simulink model "ControladorEmbebido"  (R2022b)
settings: Solver=FixedStepDiscrete  StartTime=0.0  StopTime=SIMULPARAM.T_end  FixedStep=SIMULPARAM.Ts  RelTol=1e-3  EnableMultiTasking=on
StopFcn:
  | ShowResults;
undefined symbols (not defined in the file or in its folder): ESP, IDF, IP, TCP
libraries: esp32_device_config_lib x1
Description:
  | This model is created using Waijung 2
  | (Version: 24.1a)
  | Modified using Waijung 2
  | (Version: 24.1a)
settings Model: DataDictionary=MySharedDict.sldd  SimulationMode=processor-in-the-loop (pil)  CodeVerificationMode=processor-in-the-loop (pil)  Creator=coins  LastModifiedBy=crist
settings SolverCC: AlgebraicLoopSolver=LineSearch  PositivePriorityOrder=on  AutoInsertRateTranBlk=on
settings DataIOCC: ReturnWorkspaceOutputs=off
settings OptimizationCC: EnhancedBackFolding=on  PassReuseOutputArgsAs=Individual arguments  ZeroExternalMemoryAtStartup=off  ZeroInternalMemoryAtStartup=off  OptimizeBlockOrder=speed  DifferentSizesBufferReuse=on  OptimizationCustomize=off  EfficientTunableParamExpr=on
settings DebuggingCC: ParameterTunabilityLossMsg=error  UnconnectedInputMsg=warning  UnconnectedOutputMsg=warning  UnconnectedLineMsg=warning  ModelReferenceSymbolNameMessage=none  PregeneratedLibrarySubsystemCodeDiagnostic=none  SFMachineParentedDataDiag=warning  ArithmeticOperatorsInVariantConditions=warning
settings HardwareCC: ProdBitPerPointer=32  ProdBitPerSizeT=32  ProdBitPerPtrDiffT=32  ProdLargestAtomicInteger=Long  ProdLargestAtomicFloat=Double  ProdWordSize=32  ProdHWDeviceType=Cadence Design Systems (Tensilica)->Espressif Xtensa single-/dual-core 32-bit LX6 microprocessor
settings ModelReferenceCC: UpdateModelReferenceTargets=Force  EnableRefExpFcnMdlSchedulingChecks=on  ModelReferenceNumInstancesAllowed=Single
settings SFSimCC: MATLABDynamicMemAlloc=off  CustomCodeUndefinedFunction=UseInterfaceOnly
settings RTWCC: Description=Waijung 2 ESP32 target  SystemTargetFile=esp32.tlc  TemplateMakefile=esp32.tmf  RetainRTWFile=on  CreateSILPILBlock=PIL  CodeExecutionProfiling=on  DLArmComputeVersion=19.05
settings CodeAppCC: ForceParamTrailComments=on  IgnoreCustomStorageClasses=off  OperatorAnnotations=on  SimulinkDataObjDesc=on  SFDataObjDesc=on  InsertBlockDesc=on
settings STFCustomTargetCC: TargetLangStandard=C99 (ISO)  MultiwordLength=256  ParMdlRefBuildCompliant=on  CombineOutputUpdateFcns=on  ERTCustomFileBanners=on  SupportContinuousTime=off  SupportNonInlinedSFcns=off  RemoveResetFunc=on  MATLABClassNameForMDSCustomization=Simulink.SoftwareTarget.ERTCustomization  SystemTargetFile=esp32.tlc
settings ERTTargetCC: TargetLangStandard=C99 (ISO)  CompOptLevelCompliant=off  ConcurrentExecutionCompliant=off  ModelStepFunctionPrototypeControlCompliant=off  CPPClassGenCompliant=off  UseToolchainInfoCompliant=off  ExtModeStaticAlloc=on  ExtModeStaticAllocSize=2048  ERTSrcFileBannerTemplate=esp32_code_template.cgt  ERTHdrFileBannerTemplate=esp32_code_template.cgt  ERTDataSrcFileTemplate=esp32_code_template.cgt  ERTDataHdrFileTemplate=esp32_code_template.cgt  ERTCustomFileTemplate=esp32_file_process.tlc

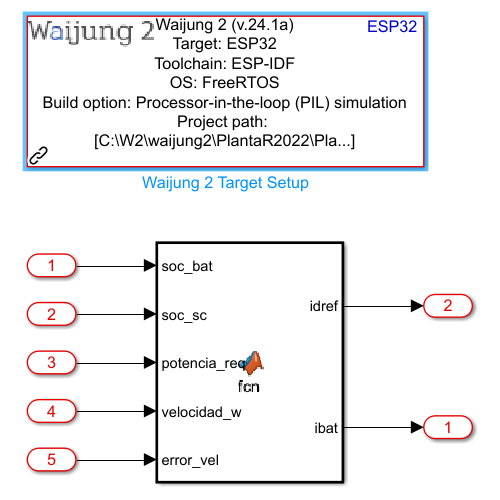
[thumbnail: Simulink's stored preview of the top-level diagram]
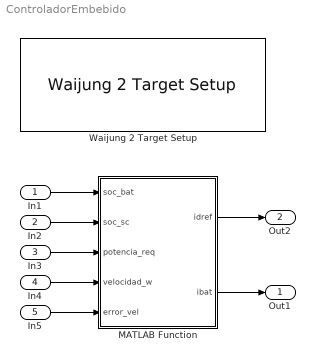
== system ControladorEmbebido ==
  In1 : Inport
  In2 : Inport  Port=2
  In3 : Inport  Port=3
  In4 : Inport  Port=4
  In5 : Inport  Port=5
  MATLAB Function : MATLAB Function  TreatAsAtomicUnit=on  SystemSampleTime=0.001
  Waijung 2 Target Setup : esp32_device_config_lib/Waijung 2 Target Setup  waijungversion=24.1a  toolchain=ESP-IDF  os=FreeRTOS  sampletime=-1  simulink_managebuildsystem=on  projectpath=C:\W2\waijung2\PlantaR2022\ControladorEmbebido_esp32_build_system  projectverprefix=waijung2  projectversuffix=1.0.0  projectversion="waijung2        1.0.0"  import_external_src=off  espidfpath=C:\msys32\home\skris\esp\esp-idf  buildoptions=Processor-in-the-loop (PIL) simulation  blockid=Waijung2TargetSetup  target=ESP32  defaultstacksize=2048  basepriority=0  highestpriority=10  generate_baserate_task=on  tickrate=1000  esp32target=ESP32  esp32targetdef=esp32  esp32flashsize=4MB  esp32comport=COM3  esp32baudrate=115200  serialmonitor=off  monitorbaudrate=115200  esp32advancedconfig=off  esp32partitiontable=Use default waijung2 partition table  esp32partitionpath=Browse the partition table  partitionname=partitions.csv  editpartition=off  custompartitiondata={'nvs','data','nvs','','0x6000','';'phy_init','data','phy','','0x1000','';'factory','app','factory','','1M',''}  reqblocks=default  esp32custompartition={'nvs','data','nvs','','0x6000','';'phy_init','data','phy','','0x1000','';'factory','app','factory','','1M',''}  cominterface=TCP/IP  uart_module=0  baudrate=115200  tx_pin=0  rx_pin=0  com_port=9  wifimode=WIFI AP  wifissid=TesisPIL  wifipassword=password  deviceip=192.168.1.10  targetgateway=192.168.1.1  targetnetmask=255.255.255.0  manualdns=on  targetdnsip=8.8.8.8  targetipport=256  targetipdef=192,168,1,10  targetmaskdef=255,255,255,0  targetgatewaydef=192,168,1,1  targetdnsipdef=8,8,8,8  hosttimeout=10  hostverbose=off
      settings: SourceProductName=Waijung 2 Blockset
  Out1 : Outport
  Out2 : Outport  Port=2
  wires:
  In2/1 -> MATLAB Function/2(soc_sc)
  MATLAB Function/1(idref) -> Out2/1
  In3/1 -> MATLAB Function/3(potencia_req)
  MATLAB Function/2(ibat) -> Out1/1
  In1/1 -> MATLAB Function/1(soc_bat)
  In4/1 -> MATLAB Function/4(velocidad_w)
  In5/1 -> MATLAB Function/5(error_vel)

== matlab function ControladorEmbebido/MATLAB Function ==
  data: idref output double; ibat output double; soc_bat input double; soc_sc input double; potencia_req input double; velocidad_w input double; error_vel input double
function [idref, ibat] = fcn(soc_bat, soc_sc, potencia_req, velocidad_w, error_vel)
%#codegen

%% --- Limitación de Entradas ---
soc_bat      = max(0, min(100, soc_bat));
soc_sc       = max(0, min(100, soc_sc));
potencia_req = max(-3.188, min(6.01308, potencia_req));
velocidad_w  = max(0, min(700, velocidad_w));
error_vel    = max(-5.25, min(5.25, error_vel));

%% --- Funciones auxiliares ---
trimf = @(x, abc) max(min((x - abc(1)) / (abc(2) - abc(1)), (abc(3) - x) / (abc(3) - abc(2))), 0) ...
                    .* double(x > abc(1) & x < abc(3));
trapmf = @(x, abcd) min(min(1, max(0, (x - abcd(1)) / (abcd(2) - abcd(1)))), ...
                        max(0, (abcd(4) - x) / (abcd(4) - abcd(3))));

%% --- Funciones de Membresía para Entradas ---
% SOC Batería
mu_soc_bat_low  = trapmf(soc_bat, [0, 0, 45, 60]);
mu_soc_bat_med  = trimf(soc_bat, [45, 60, 75]);
mu_soc_bat_high = trapmf(soc_bat, [60, 80, 100, 100]);

% SOC Supercap
mu_soc_sc_verylow = trapmf(soc_sc, [-24.894, -2.67196, 20, 40]);
mu_soc_sc_low     = trapmf(soc_sc, [10, 30, 50, 70]);
mu_soc_sc_med     = trimf(soc_sc, [50, 70, 90]);
mu_soc_sc_high    = trapmf(soc_sc, [70, 85, 102.8, 125]);

% Potencia requerida
mu_pot_baja  = trapmf(potencia_req, [-3.188, -3.17598, -1.5, 0.1875]);
mu_pot_media = trimf(potencia_req, [-1.125, 0.75, 2.625]);
mu_pot_alta  = trapmf(potencia_req, [1.312, 3, 5.09037, 6.01308]);

% Velocidad
mu_vel_nom     = trapmf(velocidad_w, [0, 0, 502.618, 510.842]);
mu_vel_baj_med = trimf(velocidad_w, [510.842, 551.963, 593.085]);
mu_vel_med     = trimf(velocidad_w, [560.188, 601.309, 642.43]);
mu_vel_med_alt = trimf(velocidad_w, [609.533, 650.654, 691.776]);
mu_vel_alta    = trimf(velocidad_w, [658.879, 700, 741.121]);

% Error de velocidad
mu_err_neg = trapmf(error_vel, [-5.25, -5.17241, -3, -0.75]);
mu_err_cer = trimf(error_vel, [-2.5, 0, 2.5]);
mu_err_pos = trapmf(error_vel, [0.75, 3, 5.24376, 5.25]);

%% --- Inicialización de Salidas y sus centroides ---
% i-bat (salida 1)
centroide_ibat = [10, 37.5, 75]; % SC, Both, Battery
acum_ibat = zeros(1, 3);

% IdRef (salida 2)
centroide_idref = [-100, -75, -50, -25, 0];
acum_idref = zeros(1, 5);

%% --- Reglas de inferencia difusa ---
% IdRef
acum_idref(5) = max(acum_idref(5), mu_vel_nom);
acum_idref(5) = max(acum_idref(5), min(mu_vel_baj_med, mu_err_pos));
acum_idref(5) = max(acum_idref(5), min(mu_vel_baj_med, mu_err_cer));
acum_idref(5) = max(acum_idref(5), min(mu_vel_baj_med, mu_err_neg));
acum_idref(4) = max(acum_idref(4), min(mu_vel_med, mu_err_pos));
acum_idref(3) = max(acum_idref(3), min(mu_vel_med, mu_err_cer));
acum_idref(2) = max(acum_idref(2), min(mu_vel_med, mu_err_neg));
acum_idref(3) = max(acum_idref(3), min(mu_vel_med_alt, mu_err_pos));
acum_idref(2) = max(acum_idref(2), min(mu_vel_med_alt, mu_err_cer));
acum_idref(1) = max(acum_idref(1), min(mu_vel_med_alt, mu_err_neg));
acum_idref(2) = max(acum_idref(2), min(mu_vel_alta, mu_err_pos));
acum_idref(1) = max(acum_idref(1), min(mu_vel_alta, mu_err_cer));
acum_idref(1) = max(acum_idref(1), min(mu_vel_alta, mu_err_neg));

% Ibat
acum_ibat(3) = max(acum_ibat(3), mu_soc_sc_low);
acum_ibat(1) = max(acum_ibat(1), min(mu_soc_sc_med, mu_pot_baja));
acum_ibat(2) = max(acum_ibat(2), mu_pot_alta); % corregido a Both
acum_ibat(3) = max(acum_ibat(3), min(mu_soc_bat_med, mu_soc_sc_low) * mu_pot_alta);
acum_ibat(3) = max(acum_ibat(3), min(mu_soc_bat_high, mu_soc_sc_low) * mu_pot_alta);
acum_ibat(2) = max(acum_ibat(2), min(mu_soc_bat_high, mu_soc_sc_med));
acum_ibat(1) = max(acum_ibat(1), min(mu_soc_bat_high, mu_soc_sc_high));
acum_ibat(1) = max(acum_ibat(1), mu_soc_sc_verylow);
acum_ibat(1) = max(acum_ibat(1), min(mu_soc_bat_low, mu_soc_sc_high) * mu_pot_media);

%% --- Desfuzzificación por Centroide ---
idref = double(0);
ibat  = double(0);

if sum(acum_idref) > 0
    idref = double(sum(acum_idref .* centroide_idref) / sum(acum_idref));
end
if sum(acum_ibat) > 0
    ibat  = double(sum(acum_ibat .* centroide_ibat) / sum(acum_ibat));
end
end
